simulink model "adcs_v15_integral_29april17"  (R2015b)
settings: Solver=ode4  StartTime=0.0  StopTime=20  FixedStep=s_SIM_STEP_SIZE  RelTol=1e-3
values from neighbouring files (symbols this model uses):
  A = ((T_SIDE + .29)*1e-3)^2    [constants_v13.m]    (also in constants_v15.m; constants_v15_Pow.m; constants_v15_Pow_ss_error.m; constants_v16_integral_kartavya.m)
  Ca_Solar_Drag = 1.4    [constants_v13.m]    (also in constants_v15.m = 0; constants_v15_Pow.m; constants_v15_Pow_ss_error.m; constants_v16_integral_kartavya.m)
  Cd = 2.2    [constants_v13.m]    (also in constants_v15.m = 0; constants_v15_Pow.m; constants_v15_Pow_ss_error.m; constants_v16_integral_kartavya.m)
  check_time = 60000    [constants_v13.m]    (also in constants_v15.m = 10000; constants_v15_Pow_ss_error.m = 10000; constants_v16_integral_kartavya.m = 10000; constants_v16_integral_light_sun_sgp_igrf_power_13Dec2011.m = 10000)
  equinox = datenum('21-Mar-2010 12:0:0')    [constants_v13.m]    (also in constants_v15.m; constants_v15_Pow.m = datenum('20-Mar-2015 12:0:0'); constants_v15_Pow_ss_error.m; constants_v16_integral_kartavya.m)
  I_MAX = 0.5    [constants_v13.m]    (also in constants_v15.m; constants_v15_Pow.m; constants_v15_Pow_ss_error.m; constants_v16_integral_kartavya.m)
  I_TORQUER = 3.6 / 7.31    (= 0.492476060192)    [constants_v13.m]    (also in constants_v15.m = 0.272727272727; constants_v15_Pow.m; constants_v15_Pow_ss_error.m; constants_v16_integral_kartavya.m)
  Kd = 2* m_INERTIA / (s_numOrbits * T_ORBIT )    [constants_v13.m]    (also in constants_v15.m = m_INERTIA * (2 + delta)* zeta * w; constants_v15_Pow.m = m_INERTIA * (2 + delta)* zeta * w; constants_v15_Pow_ss_error.m = m_INERTIA * (2 + delta)* zeta * w; constants_v16_integral_kartavya.m = m_INERTIA * (2 + delta)* zeta * w)
  Kdetumb = K_det*eye(3)    [constants_v13.m]    (also in constants_v15.m; constants_v15_Pow.m; constants_v15_Pow_ss_error.m; constants_v16_integral_kartavya.m)
  Ki = m_INERTIA * delta * zeta * w^3    [constants_v15.m]    (also in constants_v15_Pow.m; constants_v15_Pow_ss_error.m; constants_v16_integral_kartavya.m; constants_v16_integral_light_sun_sgp_igrf_power_13Dec2011.m)
  Kp = m_INERTIA / (s_numOrbits * T_ORBIT * zeta)^2    [constants_v13.m]    (also in constants_v15.m = m_INERTIA * (w*w + 2*delta*zeta^2*w^2); constants_v15_Pow.m = m_INERTIA * (w*w + 2*delta*zeta^2*w^2); constants_v15_Pow_ss_error.m = m_INERTIA * (w*w + 2*delta*zeta^2*w^2); constants_v16_integral_kartavya.m = m_INERTIA * (w*w + 2*delta*zeta^2*w^2))
  m_INERTIA = [Ixx Ixy Ixz; Ixy Iyy Iyz; Ixz Iyz Izz]    [constants_v13.m]    (also in constants_v15.m; constants_v15_Pow.m = 1*[Ixx Ixy Ixz; Ixy Iyy Iyz; Ixz Iyz Izz]; constants_v15_Pow_ss_error.m = 1*[Ixx Ixy Ixz; Ixy Iyy Iyz; Ixz Iyz Izz]; constants_v16_integral_kartavya.m)
  mu = 6.673e-11*5.9742e24    (= 398658366000000)    [constants_v13.m]    (also in constants_v15.m; constants_v15_Pow.m; constants_v15_Pow_ss_error.m; constants_v16_integral_kartavya.m)
  N = 40    [constants_v13.m]    (also in constants_v15.m = 60; constants_v15_Pow.m; constants_v15_Pow_ss_error.m; constants_v16_integral_kartavya.m)
  P_momentum_flux_from_the_sun = 4.4e-6    (= 4.4e-06)    [constants_v13.m]    (also in constants_v15.m = 0; constants_v15_Pow.m; constants_v15_Pow_ss_error.m; constants_v16_integral_kartavya.m)
  q_BI0 = x_fromEnvModel(1:4)'    [OILS_script.m]    (also in OILS_script_OBC_preflight_bounce_back.m; OILS_script_extended.m; OILS_script_preflight_test.m; constants_v13.m = euler2qBI(roll0,pitch0,yaw0))
  s_FRAME_SIZE = 2    [constants_v13.m]    (also in constants_v15.m; constants_v15_Pow.m; constants_v15_Pow_ss_error.m; constants_v16_integral_kartavya.m)
  s_m_MAX = 0.95    [constants_v13.m]    (also in constants_v15.m; constants_v15_Pow.m; constants_v15_Pow_ss_error.m; constants_v16_integral_kartavya.m)
  s_MAG_B = 2.5e-5    (= 2.5e-05)    [constants_v13.m]    (also in constants_v15.m; constants_v15_Pow.m; constants_v15_Pow_ss_error.m; constants_v16_integral_kartavya.m)
  s_MAGMETER_WEIGHT = .9    (= 0.9)    [constants_v13.m]    (also in constants_v15.m; constants_v15_Pow.m; constants_v15_Pow_ss_error.m; constants_v16_integral_kartavya.m)
  s_SIM_STEP_SIZE = 0.1    [constants_v13.m]    (also in constants_v15.m; constants_v15_Pow.m; constants_v15_Pow_ss_error.m; constants_v16_integral_kartavya.m)
  s_SS_ADC_gain = 5    [constants_v13.m]    (also in constants_v15.m = 3.3; constants_v15_Pow.m; constants_v15_Pow_ss_error.m; constants_v16_integral_kartavya.m)
  s_SS_ADC_res = 2^12 - 1    (= 4095)    [constants_v13.m]    (also in constants_v15.m = 1023; constants_v15_Pow.m; constants_v15_Pow_ss_error.m; constants_v16_integral_kartavya.m)
  s_SS_MAX_ANGLE = 85    [constants_v13.m]    (also in constants_v15.m = 55; constants_v15_Pow.m; constants_v15_Pow_ss_error.m; constants_v16_integral_kartavya.m)
  s_TAU_W = 60    [constants_v13.m]    (also in constants_v15.m; constants_v15_Pow.m; constants_v15_Pow_ss_error.m; constants_v16_integral_kartavya.m)
  s_x_MAGMETER_BIAS = 50e-9    (= 5e-08)    [constants_v13.m]    (also in constants_v15.m = 0; constants_v15_Pow.m; constants_v15_Pow_ss_error.m; constants_v16_integral_kartavya.m)
  side = 0.26    [constants_v13.m]    (also in constants_v15.m; constants_v15_Pow.m; constants_v15_Pow_ss_error.m; constants_v16_integral_kartavya.m)
  Snum = 6    [constants_v13.m]    (also in constants_v15.m; constants_v15_Pow.m; constants_v15_Pow_ss_error.m; constants_v16_integral_kartavya.m)
  TLE_epoch = datenum('18-Oct-2015 10:30:0')    [constants_v15.m]    (also in constants_v16_integral_kartavya.m = datenum('18-Oct-2010 10:30:0'); constants_v16_integral_light_sun_sgp_igrf_power_13Dec2011.m = datenum('18-Oct-2010 10:30:0'); precalcs.m)
  today = datenum('18-Oct-2010 10:30:0')    [constants_v13.m]    (also in constants_v15.m; constants_v15_Pow.m = datenum('18-Oct-2015 10:30:0'); constants_v15_Pow_ss_error.m; constants_v16_integral_kartavya.m)
  tol_q4 = 0.7    [constants_v13.m]    (also in constants_v15.m = 0.85; constants_v15_Pow.m = 0.85; constants_v15_Pow_ss_error.m = 0.85; constants_v16_integral_kartavya.m = 0.85)
  tol_w = 4e-3    (= 0.004)    [constants_v13.m]    (also in constants_v15.m; constants_v15_Pow.m; constants_v15_Pow_ss_error.m; constants_v16_integral_kartavya.m)
  tolw_n2d = 10e-3    (= 0.01)    [constants_v15.m]    (also in constants_v15_Pow.m = 0.008; constants_v15_Pow_ss_error.m; constants_v16_integral_kartavya.m; constants_v16_integral_light_sun_sgp_igrf_power_13Dec2011.m)
  Ts_display = 6    [constants_v13.m]    (also in constants_v15.m = 2; constants_v15_Pow.m; constants_v15_Pow_ss_error.m; constants_v16_integral_kartavya.m)
  v_COM_to_COP_b = [.2; 1.75; .2]*1e-2    [constants_v13.m]    (also in constants_v15.m = [.2; 1.75; .2]*0e-2; constants_v15_Pow.m; constants_v15_Pow_ss_error.m; constants_v16_integral_kartavya.m)
  v_S1 = [1 0 0]    [constants_v13.m]    (also in constants_v15.m; constants_v15_Pow.m; constants_v15_Pow_ss_error.m; constants_v16_integral_kartavya.m)
  v_S2 = [-1 0 0]    [constants_v13.m]    (also in constants_v15.m; constants_v15_Pow.m; constants_v15_Pow_ss_error.m; constants_v16_integral_kartavya.m)
  v_S3 = [0 1 0]    [constants_v13.m]    (also in constants_v15.m; constants_v15_Pow.m; constants_v15_Pow_ss_error.m; constants_v16_integral_kartavya.m)
  v_S4 = [0 -1 0]    [constants_v13.m]    (also in constants_v15.m; constants_v15_Pow.m; constants_v15_Pow_ss_error.m; constants_v16_integral_kartavya.m)
  v_S5 = [0 0 1]    [constants_v13.m]    (also in constants_v15.m; constants_v15_Pow.m; constants_v15_Pow_ss_error.m; constants_v16_integral_kartavya.m)
  v_S6 = [0 0 -1]    [constants_v13.m]    (also in constants_v15.m; constants_v15_Pow.m; constants_v15_Pow_ss_error.m; constants_v16_integral_kartavya.m)
  v_x_MOUNTING_THETA_ZYX_BODY_TORQUER = [1; 1; 1]* pi/180    [constants_v13.m]    (also in constants_v15.m; constants_v15_Pow.m; constants_v15_Pow_ss_error.m; constants_v16_integral_kartavya.m)
  wx0 = x_fromEnvModel(5)    [OILS_script.m]    (also in OILS_script_OBC_preflight_bounce_back.m; OILS_script_extended.m; OILS_script_preflight_test.m; constants_v13.m = 0.0349065850399)
  wy0 = x_fromEnvModel(6)    [OILS_script.m]    (also in OILS_script_OBC_preflight_bounce_back.m; OILS_script_extended.m; OILS_script_preflight_test.m; constants_v13.m = 0.0174532925199)
  wz0 = x_fromEnvModel(7)    [OILS_script.m]    (also in OILS_script_OBC_preflight_bounce_back.m; OILS_script_extended.m; OILS_script_preflight_test.m; constants_v13.m = -0.0349065850399)
undefined symbols (not defined in the file or in its folder): Earth, WGS84
libraries: xpcutilitieslib x17, commnoisgen2 x14, aerolibutil x2, aerolibtransform2 x1
(part 1 of 2)
settings Model: SimulationMode=accelerator  ExtModeTrigDuration=100  Creator=Jaideep  LastModifiedBy=sat_lab
settings SolverCC: AutoInsertRateTranBlk=on
settings DataIOCC: ExternalInput=constants_v13  SaveFinalState=on  SaveFormat=Array  SignalLoggingSaveFormat=ModelDataLogs  SaveOutput=off  SaveState=on  StateSaveName=tmp_raccel_xout
settings OptimizationCC: ExpressionDepthLimit=2147483647  EfficientMapNaN2IntZero=off
settings DebuggingCC: UnderspecifiedInitializationDetection=Classic  MergeDetectMultiDrivingBlocksExec=none  SolverPrmCheckMsg=warning  FcnCallInpInsideContextMsg=UseLocalSettings  StateNameClashWarn=warning
settings HardwareCC: ProdBitPerPointer=32  ProdLargestAtomicFloat=None  ProdIntDivRoundTo=Undefined  ProdEndianess=Unspecified  ProdWordSize=32  ProdHWDeviceType=32-bit Generic  TargetBitPerPointer=64  TargetLongLongMode=on  TargetIntDivRoundTo=Zero  TargetEndianess=LittleEndian  TargetWordSize=64  TargetHWDeviceType=MATLAB Host  ProdEqTarget=off
settings SFSimCC: SimParseCustomCode=off
settings RTWCC: SystemTargetFile=raccel.tlc  TemplateMakefile=raccel_default_tmf  RTWVerbose=off
settings CodeAppCC: GenerateComments=off  MaxIdLength=128  SimulinkBlockComments=off
settings RaccelTargetCC: ERTMultiwordTypeDef=System defined  ERTMultiwordLength=256  ParMdlRefBuildCompliant=off  GeneratePreprocessorConditionals=Disable all  ERTFirstTimeCompliant=off  MultiInstanceERTCode=off  ENABLE_SLEXEC_SSBRIDGE=0  RTWCAPIParams=on
settings ConfigComp: CovModelRefEnable=Off

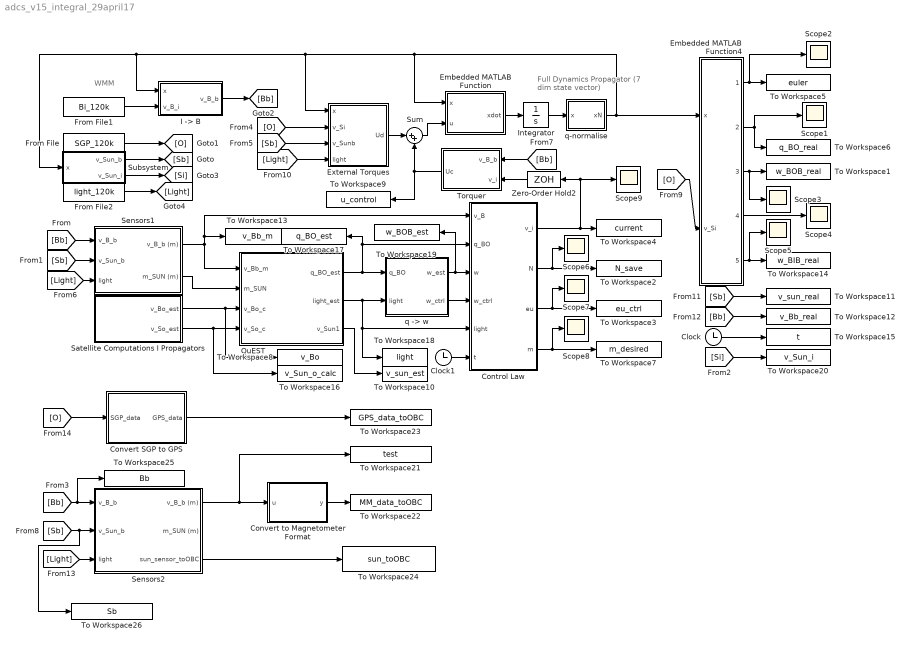
== system adcs_v15_integral_29april17 ==
  note: Full Dynamics Propagator
      |  (7 dim state vector)
  note: WMM
  Clock : Clock
  Clock1 : Clock
  Control Law : Subsystem  TreatAsAtomicUnit=on  SystemSampleTime=s_FRAME_SIZE
  Convert SGP to GPS : Subsystem
  Convert to Magnetometer Format : MATLAB Function  TreatAsAtomicUnit=on
  Embedded MATLAB Function : MATLAB Function  TreatAsAtomicUnit=on
  Embedded MATLAB Function4 : MATLAB Function  TreatAsAtomicUnit=on
  External Torques : Subsystem
  From File : FromFile  FileName=SGP_120k
  From File1 : FromFile  FileName=Bi_120k
  From File2 : FromFile  FileName=light_120k  SampleTime=0
  "I -> B" : Subsystem
  Integrator : Integrator  InitialCondition=[q_BI0; wx0; wy0; wz0]
  QuEST : MATLAB Function  TreatAsAtomicUnit=on  SystemSampleTime=s_FRAME_SIZE
  Satellite Computations I Propagators : Subsystem  TreatAsAtomicUnit=on  SystemSampleTime=s_FRAME_SIZE
  Scope{1..9} (9 alike) : Scope
  Sensors1 : Subsystem
  Sensors2 : Subsystem
  Subsystem : Subsystem
  Sum : Sum  Inputs=|++
  To Workspace1 : ToWorkspace  VariableName=w_BOB_real  SampleTime=Ts_display
  To Workspace10 : ToWorkspace  VariableName=v_sun_est  SampleTime=Ts_display
  To Workspace11 : ToWorkspace  VariableName=v_sun_real  SampleTime=Ts_display
  To Workspace12 : ToWorkspace  VariableName=v_Bb_real  SampleTime=Ts_display
  To Workspace13 : ToWorkspace  VariableName=v_Bb_m  SampleTime=Ts_display
  To Workspace14 : ToWorkspace  VariableName=w_BIB_real  SampleTime=Ts_display
  To Workspace15 : ToWorkspace  VariableName=t  SampleTime=Ts_display
  To Workspace16 : ToWorkspace  VariableName=v_Sun_o_calc  SampleTime=Ts_display
  To Workspace17 : ToWorkspace  VariableName=q_BO_est  SampleTime=Ts_display
  To Workspace18 : ToWorkspace  VariableName=light  SampleTime=Ts_display
  To Workspace19 : ToWorkspace  VariableName=w_BOB_est  SampleTime=Ts_display
  To Workspace2 : ToWorkspace  VariableName=N_save  SampleTime=Ts_display
  To Workspace20 : ToWorkspace  VariableName=v_Sun_i  SampleTime=Ts_display
  To Workspace21 : ToWorkspace  VariableName=test  SampleTime=-1
  To Workspace22 : ToWorkspace  VariableName=MM_data_toOBC  SampleTime=Ts_display
  To Workspace23 : ToWorkspace  VariableName=GPS_data_toOBC  SampleTime=Ts_display
  To Workspace24 : ToWorkspace  VariableName=sun_toOBC  SampleTime=Ts_display
  To Workspace25 : ToWorkspace  VariableName=Bb  SampleTime=-1
  To Workspace26 : ToWorkspace  VariableName=Sb  SampleTime=-1
  To Workspace3 : ToWorkspace  VariableName=eu_ctrl  SampleTime=Ts_display
  To Workspace4 : ToWorkspace  VariableName=current  SampleTime=Ts_display
  To Workspace5 : ToWorkspace  VariableName=euler  SampleTime=Ts_display
  To Workspace6 : ToWorkspace  VariableName=q_BO_real  SampleTime=Ts_display
  To Workspace7 : ToWorkspace  VariableName=m_desired  SampleTime=Ts_display
  To Workspace8 : ToWorkspace  VariableName=v_Bo  SampleTime=Ts_display
  To Workspace9 : ToWorkspace  VariableName=u_control  SampleTime=Ts_display
  Torquer : Subsystem
  Zero-Order Hold2 : ZeroOrderHold  SampleTime=s_FRAME_SIZE
  "q -> w" : Subsystem  TreatAsAtomicUnit=on  SystemSampleTime=s_FRAME_SIZE
  q-normalise : MATLAB Function  TreatAsAtomicUnit=on
  wires:
  Embedded MATLAB Function/1(xdot) -> Integrator/1
  Integrator/1 -> q-normalise/1(x)
  From File/1 -> [O]
  q-normalise/1(xN) -> Subsystem/1(x), "I -> B"/1(x), External Torques/1(x), Embedded MATLAB Function/1(x), Embedded MATLAB Function4/1(x)
  Sum/1 -> Embedded MATLAB Function/2(u)
  "I -> B"/1(v_B_b) -> [Bb]
  Subsystem/1(v_Sun_b) -> [Sb]
  [Bb] -> Sensors1/1(v_B_b)
  [Sb] -> Sensors1/2(v_Sun_b)
  Subsystem/2(v_Sun_i) -> [Si]
  [O] -> External Torques/2(v_Si)
  [Sb] -> External Torques/3(v_Sunb)
  [Bb] -> Torquer/1(v_B_b)
  [Light] -> Sensors1/3(light)
  Sensors1/2(m_SUN (m)) -> QuEST/2(m_SUN)
  Sensors1/1(v_B_b (m)) -> QuEST/1(v_Bb_m), Control Law/1(v_B), To Workspace13/1
  Zero-Order Hold2/1 -> Torquer/2(v_i)
  Torquer/1(Uc) -> Sum/2, To Workspace9/1
  Satellite Computations I Propagators/1(v_Bo_est) -> To Workspace8/1, QuEST/3(v_Bo_c)
  Satellite Computations I Propagators/2(v_So_est) -> To Workspace16/1, QuEST/4(v_So_c)
  QuEST/1(q_BO_est) -> "q -> w"/1(q_BO), Control Law/2(q_BO), To Workspace17/1
  QuEST/2(light_est) -> "q -> w"/2(light), Control Law/5(light), To Workspace18/1
  Control Law/1(v_i) -> To Workspace4/1, Zero-Order Hold2/1, Scope9/1
  [O] -> Embedded MATLAB Function4/2(v_Si)
  Control Law/2(N) -> To Workspace2/1, Scope6/1
  From File2/1 -> [Light]
  Control Law/3(eu) -> To Workspace3/1, Scope7/1
  Control Law/4(m) -> To Workspace7/1, Scope8/1
  "q -> w"/1(w_est) -> Control Law/3(w), To Workspace19/1
  [Light] -> External Torques/4(light)
  "q -> w"/2(w_ctrl) -> Control Law/4(w_ctrl)
  QuEST/3(v_Sun1) -> To Workspace10/1
  [Sb] -> To Workspace11/1
  [Bb] -> To Workspace12/1
  Clock/1 -> To Workspace15/1
  From File1/1 -> "I -> B"/2(v_B_i)
  Clock1/1 -> Control Law/6(t)
  Embedded MATLAB Function4/3(w_BOB) -> To Workspace1/1, Scope3/1
  Embedded MATLAB Function4/2(q_BO) -> To Workspace6/1, Scope1/1
  Embedded MATLAB Function4/1(euler) -> To Workspace5/1, Scope2/1
  Embedded MATLAB Function4/5(w_BIB) -> To Workspace14/1, Scope5/1
  Embedded MATLAB Function4/4(modw) -> Scope4/1
  [Si] -> To Workspace20/1
  External Torques/1(Ud) -> Sum/1
  [O] -> Convert SGP to GPS/1(SGP_data)
  Convert SGP to GPS/1(GPS_data) -> To Workspace23/1
  Convert to Magnetometer Format/1(y) -> To Workspace22/1
  [Bb] -> To Workspace25/1, Sensors2/1(v_B_b)
  [Sb] -> To Workspace26/1, Sensors2/2(v_Sun_b)
  [Light] -> Sensors2/3(light)
  Sensors2/3(sun_sensor_toOBC) -> To Workspace24/1
  Sensors2/1(v_B_b (m)) -> To Workspace21/1, Convert to Magnetometer Format/1(u)

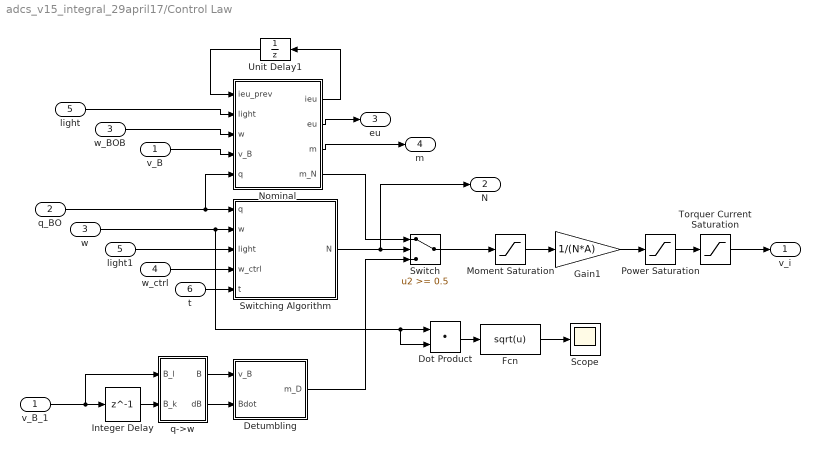
== system adcs_v15_integral_29april17/Control Law ==
  v_B : Inport
  q_BO : Inport  Port=2
  w : Inport  Port=3
  w_ctrl : Inport  Port=4
  light : Inport  Port=5
  t : Inport  Port=6
  Detumbling : MATLAB Function  TreatAsAtomicUnit=on
  Dot Product : DotProduct  InputSameDT=on  OutDataTypeStr=Inherit: Inherit via internal rule
  Fcn : Fcn  Expr=sqrt(u)
  Gain1 : Gain  Gain=1/(N*A)
  Integer Delay : Delay  DelayLength=1  InputProcessing=Inherited
  Moment Saturation : Saturate  UpperLimit=s_m_MAX  LowerLimit=-s_m_MAX
  Nominal : MATLAB Function  TreatAsAtomicUnit=on
  Power Saturation : Saturate  UpperLimit=I_MAX  LowerLimit=-I_MAX
  Scope : Scope
  Switch : Switch  Threshold=0.5
  Switching Algorithm : Subsystem
  Torquer Current Saturation : Saturate  UpperLimit=I_TORQUER  LowerLimit=-I_TORQUER
  Unit Delay1 : UnitDelay  InitialCondition=[0;0;0]  SampleTime=-1
  light1 : InportShadow  Port=5
  q->w : MATLAB Function  TreatAsAtomicUnit=on
  v_B_1 : InportShadow
  w_BOB : InportShadow  Port=3
  v_i : Outport
  N : Outport  Port=2
  eu : Outport  Port=3
  m : Outport  Port=4
  wires:
  w_ctrl/1 -> Switching Algorithm/4(w_ctrl)
  Nominal/3(m) -> m/1
  Nominal/2(eu) -> eu/1
  w_BOB/1 -> Nominal/3(w)
  light1/1 -> Switching Algorithm/3(light)
  v_B/1 -> Nominal/4(v_B)
  q->w/2(dB) -> Detumbling/2(Bdot)
  v_B_1/1 -> Integer Delay/1, q->w/1(B_l)
  w/1 -> Switching Algorithm/2(w), Dot Product/1, Dot Product/2
  Nominal/4(m_N) -> Switch/1
  Switching Algorithm/1(N) -> Switch/2, N/1
  Detumbling/1(m_D) -> Switch/3
  Switch/1 -> Moment Saturation/1
  Power Saturation/1 -> Torquer Current Saturation/1
  Moment Saturation/1 -> Gain1/1
  Torquer Current Saturation/1 -> v_i/1
  Gain1/1 -> Power Saturation/1
  light/1 -> Nominal/2(light)
  q_BO/1 -> Switching Algorithm/1(q), Nominal/5(q)
  Integer Delay/1 -> q->w/2(B_k)
  q->w/1(B) -> Detumbling/1(v_B)
  t/1 -> Switching Algorithm/5(t)
  Dot Product/1 -> Fcn/1
  Fcn/1 -> Scope/1
  Unit Delay1/1 -> Nominal/1(ieu_prev)
  Nominal/1(ieu) -> Unit Delay1/1

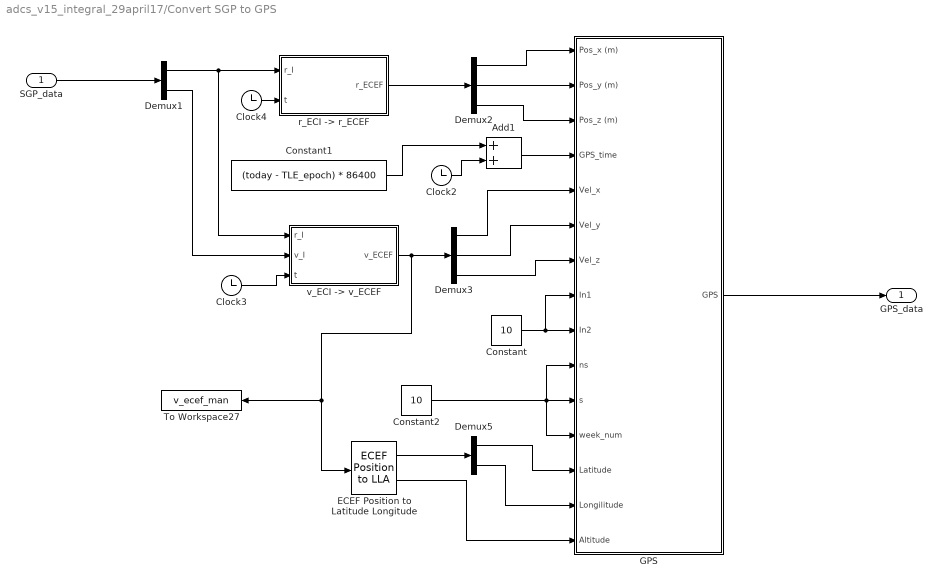
== system adcs_v15_integral_29april17/Convert SGP to GPS ==
  SGP_data : Inport
  Add1 : Sum
  Clock2 : Clock
  Clock3 : Clock
  Clock4 : Clock
  Constant : Constant  Value=10  OutDataTypeStr=uint8
  Constant1 : Constant  Value=(today - TLE_epoch) * 86400  VectorParams1D=off
  Constant2 : Constant  Value=10  OutDataTypeStr=double
  Demux1 : Demux  Outputs=2
  Demux2 : Demux  Outputs=3
  Demux3 : Demux  Outputs=3
  Demux5 : Demux  Outputs=2
  ECEF Position to Latitude Longitude : aerolibtransform2/ECEF Position to LLA  units=Metric (MKS)  ptype=Earth (WGS84)  F=1/298.257223563  R=6378137
  GPS : Subsystem
  To Workspace27 : ToWorkspace  VariableName=v_ecef_man  SampleTime=Ts_display
  "r_ECI -> r_ECEF" : MATLAB Function  TreatAsAtomicUnit=on
  "v_ECI -> v_ECEF" : MATLAB Function  TreatAsAtomicUnit=on
  GPS_data : Outport
  wires:
  Constant/1 -> GPS/9(In2), GPS/8(In1)
  ECEF Position to Latitude Longitude/1 -> Demux5/1
  ECEF Position to Latitude Longitude/2 -> GPS/15(Altitude)
  Constant2/1 -> GPS/10(ns), GPS/12(week_num), GPS/11(s)
  Demux5/1 -> GPS/13(Latitude)
  GPS/1(GPS) -> GPS_data/1
  Demux5/2 -> GPS/14("Longilitude ")
  Constant1/1 -> Add1/1
  Clock2/1 -> Add1/2
  Add1/1 -> GPS/4(GPS_time)
  Demux1/2 -> "v_ECI -> v_ECEF"/2(v_I)
  "v_ECI -> v_ECEF"/1(v_ECEF) -> Demux3/1, ECEF Position to Latitude Longitude/1, To Workspace27/1
  Demux3/1 -> GPS/5(Vel_x)
  Demux3/2 -> GPS/6(Vel_y)
  Clock3/1 -> "v_ECI -> v_ECEF"/3(t)
  Demux3/3 -> GPS/7(Vel_z)
  "r_ECI -> r_ECEF"/1(r_ECEF) -> Demux2/1
  Demux2/1 -> GPS/1(Pos_x (m))
  Demux2/2 -> GPS/2(Pos_y (m))
  Demux2/3 -> GPS/3(Pos_z (m))
  Demux1/1 -> "v_ECI -> v_ECEF"/1(r_I), "r_ECI -> r_ECEF"/1(r_I)
  SGP_data/1 -> Demux1/1
  Clock4/1 -> "r_ECI -> r_ECEF"/2(t)

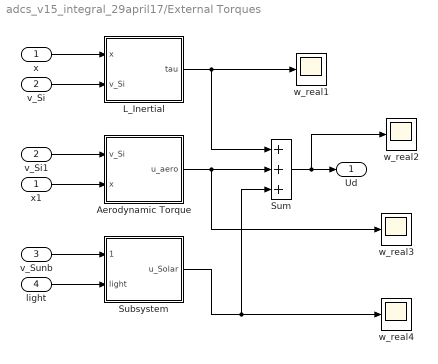
== system adcs_v15_integral_29april17/External Torques ==
  x : Inport
  v_Si : Inport  Port=2
  v_Sunb : Inport  Port=3
  light : Inport  Port=4
  Aerodynamic Torque : Subsystem
  L_Inertial : MATLAB Function  TreatAsAtomicUnit=on
  Subsystem : Subsystem
  Sum : Sum  Inputs=+++
  v_Si1 : InportShadow  Port=2
  w_real{1..4} (4 alike) : Scope
  x1 : InportShadow
  Ud : Outport
  wires:
  x/1 -> L_Inertial/1(x)
  v_Si/1 -> L_Inertial/2(v_Si)
  L_Inertial/1(tau) -> Sum/1, w_real1/1
  Aerodynamic Torque/1(u_aero) -> Sum/2, w_real3/1
  x1/1 -> Aerodynamic Torque/2(x)
  v_Si1/1 -> Aerodynamic Torque/1(v_Si)
  Sum/1 -> Ud/1, w_real2/1
  v_Sunb/1 -> Subsystem/1(v_Sun_b)
  Subsystem/1(u_Solar) -> Sum/3, w_real4/1
  light/1 -> Subsystem/2(light)

== system adcs_v15_integral_29april17/I -> B ==
  x : Inport
  v_B_i : Inport  Port=2
  Gain : Gain  Gain=1e-9
  L_Inertial : MATLAB Function  TreatAsAtomicUnit=on
  v_B_b : Outport
  wires:
  L_Inertial/1(v_B) -> v_B_b/1
  x/1 -> L_Inertial/1(x)
  v_B_i/1 -> Gain/1
  Gain/1 -> L_Inertial/2(v_I)

== system adcs_v15_integral_29april17/Satellite Computations I Propagators ==
  From File : FromFile  FileName=Si_120k
  From File2 : FromFile  FileName=SGP_est_120k
  From File3 : FromFile  FileName=Bi8_est_120k
  m_TOI_NEW : MATLAB Function  TreatAsAtomicUnit=on
  m_TOI_NEW1 : MATLAB Function  TreatAsAtomicUnit=on
  v_Bo_est : Outport
  v_So_est : Outport  Port=2
  wires:
  From File3/1 -> m_TOI_NEW/2(v_I)
  From File2/1 -> m_TOI_NEW1/2(ECI), m_TOI_NEW/1(ECI)
  From File/1 -> m_TOI_NEW1/1(v_I)
  m_TOI_NEW/1(v_O) -> v_Bo_est/1
  m_TOI_NEW1/1(v_O) -> v_So_est/1

== system adcs_v15_integral_29april17/Sensors1 ==
  note: 'm' stands for measured
  v_B_b : Inport
  v_Sun_b : Inport  Port=2
  light : Inport  Port=3
  Magnetometer simple : Subsystem
  Sun Sensors : Subsystem
  v_B_b (m) : Outport
  m_SUN (m) : Outport  Port=2
  wires:
  light/1 -> Sun Sensors/2(Light)
  Magnetometer simple/1(v_B_b(m)) -> v_B_b (m)/1
  v_B_b/1 -> Magnetometer simple/1(v_B_b)
  v_Sun_b/1 -> Sun Sensors/1(v_Sun_b)
  Sun Sensors/1(m_SUN) -> m_SUN (m)/1

== system adcs_v15_integral_29april17/Sensors2 ==
  note: 'm' stands for measured
  v_B_b : Inport
  v_Sun_b : Inport  Port=2
  light : Inport  Port=3
  Magnetometer simple : Subsystem
  Sun Sensors : Subsystem
  v_B_b (m) : Outport
  m_SUN (m) : Outport  Port=2
  sun_sensor_toOBC : Outport  Port=3
  wires:
  light/1 -> Sun Sensors/2(Light)
  Magnetometer simple/1(v_B_b(m)) -> v_B_b (m)/1
  v_B_b/1 -> Magnetometer simple/1(v_B_b)
  v_Sun_b/1 -> Sun Sensors/1(v_Sun_b)
  Sun Sensors/1(m_SUN) -> m_SUN (m)/1
  Sun Sensors/2(sun_sensor_toOBC) -> sun_sensor_toOBC/1

== system adcs_v15_integral_29april17/Subsystem ==
  x : Inport
  From File : FromFile  FileName=Si_120k  SampleTime=0
  f: I->B : MATLAB Function  TreatAsAtomicUnit=on
  v_Sun_b : Outport
  v_Sun_i : Outport  Port=2
  wires:
  x/1 -> f: I->B/1(x)
  f: I->B/1(v_B) -> v_Sun_b/1
  From File/1 -> f: I->B/2(v_I), v_Sun_i/1

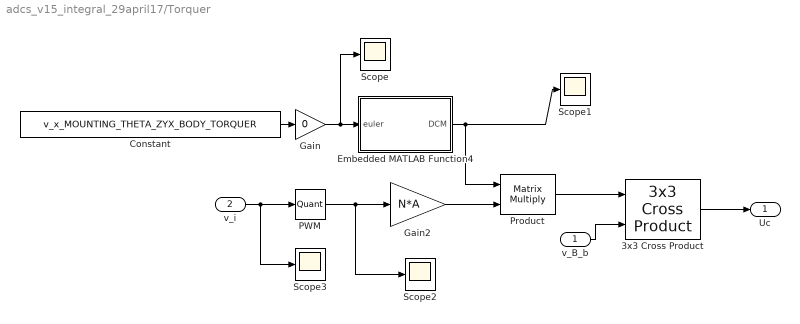
== system adcs_v15_integral_29april17/Torquer ==
  v_B_b : Inport
  v_i : Inport  Port=2
  3x3 Cross Product : aerolibutil/3x3 Cross Product
  Constant : Constant  Value=v_x_MOUNTING_THETA_ZYX_BODY_TORQUER
  Embedded MATLAB Function4 : MATLAB Function  TreatAsAtomicUnit=on
  Gain : Gain  Gain=0
  Gain2 : Gain  Gain=N*A
  PWM : Quantizer  QuantizationInterval=s_PWM_RES
  Product : Product  Multiplication=Matrix(*)  RndMeth=Zero
  Scope{,1..3} (4 alike) : Scope
  Uc : Outport
  wires:
  PWM/1 -> Gain2/1, Scope2/1
  v_B_b/1 -> 3x3 Cross Product/2
  3x3 Cross Product/1 -> Uc/1
  v_i/1 -> PWM/1, Scope3/1
  Embedded MATLAB Function4/1(DCM) -> Product/1, Scope1/1
  Gain2/1 -> Product/2
  Product/1 -> 3x3 Cross Product/1
  Constant/1 -> Gain/1
  Gain/1 -> Embedded MATLAB Function4/1(euler), Scope/1

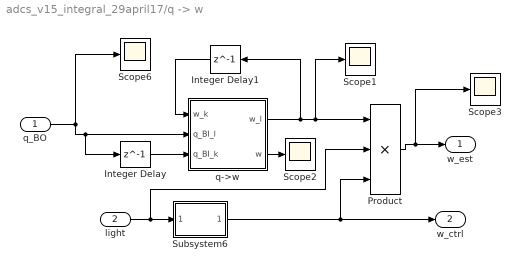
== system adcs_v15_integral_29april17/q -> w ==
  q_BO : Inport
  light : Inport  Port=2
  Integer Delay : Delay  DelayLength=1  InputProcessing=Inherited
  Integer Delay1 : Delay  DelayLength=1  InitialCondition=[0;0;0]  InputProcessing=Inherited
  Product : Product  Inputs=3  RndMeth=Zero
  Scope{1..3,6} (4 alike) : Scope
  Subsystem6 : Subsystem
  q->w : MATLAB Function  TreatAsAtomicUnit=on
  w_est : Outport
  w_ctrl : Outport  Port=2
  wires:
  Subsystem6/1(w-ctrl) -> w_ctrl/1, Product/3
  q_BO/1 -> Integer Delay/1, q->w/2(q_BI_l), Scope6/1
  light/1 -> Product/2, Subsystem6/1(light)
  Product/1 -> w_est/1, Scope3/1
  Integer Delay/1 -> q->w/3(q_BI_k)
  q->w/1(w_l) -> Integer Delay1/1, Product/1, Scope1/1
  Integer Delay1/1 -> q->w/1(w_k)
  q->w/2(w) -> Scope2/1

== system adcs_v15_integral_29april17/Control Law/Switching Algorithm ==
  note: remov the t=0 checking
      | code, not necessary
  q : Inport
  w : Inport  Port=2
  light : Inport  Port=3
  w_ctrl : Inport  Port=4
  t : Inport  Port=5
  Scope1 : Scope
  Unit Delay : UnitDelay  SampleTime=-1
  Unit Delay1 : UnitDelay  SampleTime=-1
  gate pulse : MATLAB Function  TreatAsAtomicUnit=on
  N : Outport
  wires:
  t/1 -> gate pulse/4(t)
  w_ctrl/1 -> gate pulse/6(w_ctrl)
  light/1 -> gate pulse/5(light_flag)
  gate pulse/1(N) -> N/1, Unit Delay1/1
  q/1 -> gate pulse/3(q)
  gate pulse/3(t_now) -> Unit Delay/1
  w/1 -> gate pulse/2(w)
  Unit Delay/1 -> gate pulse/7(t_now_prev)
  Unit Delay1/1 -> gate pulse/1(N_prev)
  gate pulse/2(P) -> Scope1/1

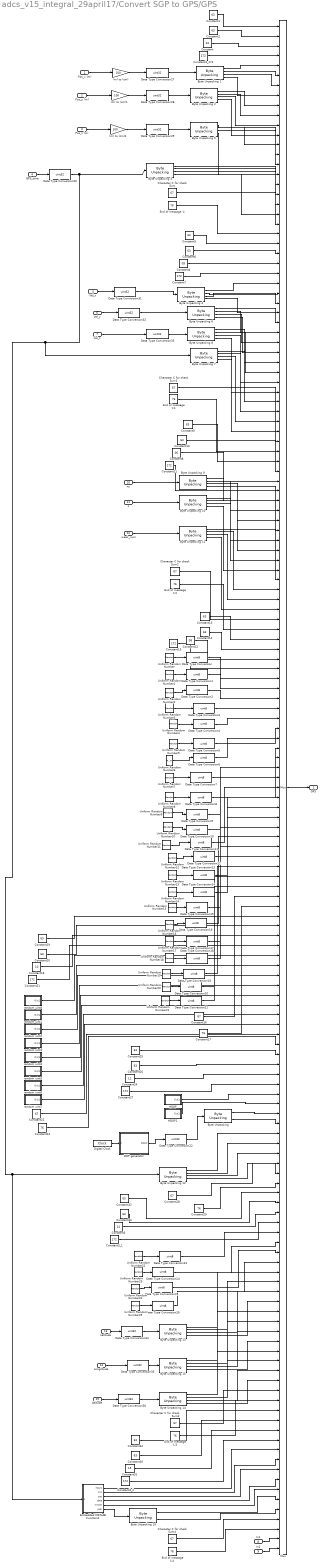
== system adcs_v15_integral_29april17/Convert SGP to GPS/GPS ==
  Pos_x (m) : Inport
  Pos_y (m) : Inport  Port=2
  Pos_z (m) : Inport  Port=3
  GPS_time : Inport  Port=4
  Vel_x : Inport  Port=5
  Vel_y : Inport  Port=6
  Vel_z : Inport  Port=7
  In1 : Inport  Port=8  OutDataTypeStr=uint8
  In2 : Inport  Port=9  OutDataTypeStr=uint8
  ns : Inport  Port=10
  s : Inport  Port=11
  week_num : Inport  Port=12
  Latitude : Inport  Port=13
  "Longilitude " : Inport  Port=14
  Altitude : Inport  Port=15
  (m) to (cm) : Gain  Gain=100  OutDataTypeStr=double
  (m) to (cm)1 : Gain  Gain=100
  (m) to (cm)2 : Gain  Gain=100
  Byte Unpacking {,1..16} (17 alike) : xpcutilitieslib/Byte Unpacking 
  Character C for check Sum{,1..4} (5 alike) : Constant  Value=67  OutDataTypeStr=uint8
  Constant : Constant  Value=04  OutDataTypeStr=uint8
  Constant{1..2,5..6,9..10,13..14,19..20,25..26,32..35} (16 alike) : Constant  Value=63  OutDataTypeStr=uint8
  Constant{7,11,15,21,27} (5 alike) : Constant  Value=172  OutDataTypeStr=uint8
  Constant12 : Constant  Value=08  OutDataTypeStr=uint8
  Constant16 : Constant  Value=67  OutDataTypeStr=uint8
  Constant17 : Constant  Value=76  OutDataTypeStr=uint8
  Constant18 : Constant  Value=10  OutDataTypeStr=uint8
  Constant22 : Constant  Value=67  OutDataTypeStr=uint8
  Constant23 : Constant  Value=76  OutDataTypeStr=uint8
  Constant24 : Constant  Value=11  OutDataTypeStr=uint8
  Constant28 : Constant  Value=67  OutDataTypeStr=uint8
  Constant29 : Constant  Value=76  OutDataTypeStr=uint8
  Constant3 : Constant  Value=14  OutDataTypeStr=uint8
  Constant31 : Constant  Value=15  OutDataTypeStr=uint8
  Constant3_1 : Constant  Value=172  OutDataTypeStr=uint8
  Constant3_172 : Constant  Value=172  OutDataTypeStr=uint8
  Constant3_2 : Constant  Value=172  OutDataTypeStr=uint8
  Constant4 : Constant  Value=05  OutDataTypeStr=uint8
  Constant8 : Constant  Value=06  OutDataTypeStr=uint8
  DOP generator : MATLAB Function  TreatAsAtomicUnit=on
  Data Type Conversion{,1..21,23..26} (26 alike) : DataTypeConversion  OutDataTypeStr=uint8
  Data Type Conversion{22,27..36} (11 alike) : DataTypeConversion  OutDataTypeStr=uint32
  Digital Clock : DigitalClock  SampleTime=0.1
  Embedded MATLAB Function2 : MATLAB Function  TreatAsAtomicUnit=on
  End of message 'L'{,1..4} (5 alike) : Constant  Value=76  OutDataTypeStr=uint8
  HDOP : Subsystem
  HDOP1 : Subsystem
  Mux : Mux  Inputs=155
  Uniform Random Number{,1..25} (26 alike) : UniformRandomNumber  Minimum=0  Maximum=256  Seed=1  SampleTime=0.1
  random uint1 : Subsystem
  random uint2 : Subsystem
  random uint3 : Subsystem
  random uint4 : Subsystem
  random uint5 : Subsystem
  random uint6 : Subsystem
  random uint7 : Subsystem
  random uint8 : Subsystem
  GPS : Outport
  wires:
  Constant1/1 -> Mux/1
  Constant2/1 -> Mux/2
  Constant/1 -> Mux/3
  Constant3_172/1 -> Mux/4
  GPS_time/1 -> Data Type Conversion30/1
  Byte Unpacking 3/1 -> Mux/17
  Byte Unpacking 3/2 -> Mux/18
  Byte Unpacking 3/3 -> Mux/19
  Character C for check Sum/1 -> Mux/21
  End of message 'L'/1 -> Mux/22
  Byte Unpacking 3/4 -> Mux/20
  Pos_x (m)/1 -> (m) to (cm)/1
  Pos_y (m)/1 -> (m) to (cm)1/1
  Pos_z (m)/1 -> (m) to (cm)2/1
  Byte Unpacking 5/1 -> Mux/13
  Byte Unpacking 5/2 -> Mux/14
  Byte Unpacking 5/3 -> Mux/15
  Byte Unpacking 5/4 -> Mux/16
  Byte Unpacking 1/1 -> Mux/5
  Byte Unpacking 1/2 -> Mux/6
  Byte Unpacking 1/3 -> Mux/7
  Byte Unpacking 1/4 -> Mux/8
  Byte Unpacking 2/1 -> Mux/9
  Byte Unpacking 2/2 -> Mux/10
  Byte Unpacking 2/3 -> Mux/11
  Byte Unpacking 2/4 -> Mux/12
  Constant5/1 -> Mux/23
  Constant6/1 -> Mux/24
  Constant4/1 -> Mux/25
  Constant7/1 -> Mux/26
  Byte Unpacking 4/1 -> Mux/27
  Byte Unpacking 4/2 -> Mux/28
  Byte Unpacking 4/3 -> Mux/29
  Byte Unpacking 4/4 -> Mux/30
  Byte Unpacking 6/1 -> Mux/31
  Byte Unpacking 6/2 -> Mux/32
  Byte Unpacking 6/3 -> Mux/33
  Byte Unpacking 6/4 -> Mux/34
  Byte Unpacking 8/1 -> Mux/35
  Byte Unpacking 8/2 -> Mux/36
  Byte Unpacking 8/3 -> Mux/37
  Byte Unpacking 8/4 -> Mux/38
  Byte Unpacking 7/1 -> Mux/39
  Byte Unpacking 7/2 -> Mux/40
  Byte Unpacking 7/3 -> Mux/41
  Byte Unpacking 7/4 -> Mux/42
  Character C for check Sum1/1 -> Mux/43
  End of message 'L'1/1 -> Mux/44
  Constant9/1 -> Mux/45
  Constant10/1 -> Mux/46
  Constant8/1 -> Mux/47
  Constant11/1 -> Mux/48
  Byte Unpacking 9/1 -> Mux/49
  Byte Unpacking 9/2 -> Mux/50
  Byte Unpacking 9/3 -> Mux/51
  Byte Unpacking 9/4 -> Mux/52
  Byte Unpacking 10/1 -> Mux/53
  Byte Unpacking 10/2 -> Mux/54
  Byte Unpacking 10/3 -> Mux/55
  Byte Unpacking 10/4 -> Mux/56
  Byte Unpacking 11/1 -> Mux/57
  Byte Unpacking 11/2 -> Mux/58
  Byte Unpacking 11/3 -> Mux/59
  Byte Unpacking 11/4 -> Mux/60
  Character C for check Sum2/1 -> Mux/61
  End of message 'L'2/1 -> Mux/62
  Uniform Random Number/1 -> Data Type Conversion/1
  Uniform Random Number1/1 -> Data Type Conversion1/1
  Uniform Random Number2/1 -> Data Type Conversion2/1
  Uniform Random Number3/1 -> Data Type Conversion3/1
  Uniform Random Number4/1 -> Data Type Conversion4/1
  Uniform Random Number5/1 -> Data Type Conversion5/1
  Uniform Random Number6/1 -> Data Type Conversion6/1
  Uniform Random Number7/1 -> Data Type Conversion7/1
  Uniform Random Number8/1 -> Data Type Conversion8/1
  Uniform Random Number9/1 -> Data Type Conversion9/1
  Uniform Random Number10/1 -> Data Type Conversion10/1
  Uniform Random Number11/1 -> Data Type Conversion11/1
  Uniform Random Number12/1 -> Data Type Conversion12/1
  Uniform Random Number13/1 -> Data Type Conversion13/1
  Uniform Random Number14/1 -> Data Type Conversion14/1
  Uniform Random Number15/1 -> Data Type Conversion15/1
  Uniform Random Number16/1 -> Data Type Conversion16/1
  Uniform Random Number17/1 -> Data Type Conversion17/1
  Uniform Random Number18/1 -> Data Type Conversion18/1
  Uniform Random Number19/1 -> Data Type Conversion19/1
  Uniform Random Number20/1 -> Data Type Conversion20/1
  Uniform Random Number21/1 -> Data Type Conversion21/1
  Constant13/1 -> Mux/63
  Constant14/1 -> Mux/64
  Constant12/1 -> Mux/65
  Constant15/1 -> Mux/66
  Data Type Conversion/1 -> Mux/67
  Data Type Conversion1/1 -> Mux/68
  Data Type Conversion2/1 -> Mux/69
  Data Type Conversion3/1 -> Mux/70
  Data Type Conversion4/1 -> Mux/71
  Data Type Conversion5/1 -> Mux/72
  Data Type Conversion6/1 -> Mux/73
  Data Type Conversion7/1 -> Mux/74
  Data Type Conversion8/1 -> Mux/75
  Data Type Conversion9/1 -> Mux/76
  Data Type Conversion10/1 -> Mux/77
  Data Type Conversion11/1 -> Mux/78
  Data Type Conversion12/1 -> Mux/79
  Data Type Conversion13/1 -> Mux/80
  Data Type Conversion14/1 -> Mux/81
  Data Type Conversion15/1 -> Mux/82
  Data Type Conversion16/1 -> Mux/83
  Data Type Conversion17/1 -> Mux/84
  Data Type Conversion18/1 -> Mux/85
  Data Type Conversion19/1 -> Mux/86
  Data Type Conversion20/1 -> Mux/87
  Data Type Conversion21/1 -> Mux/88
  Constant16/1 -> Mux/89
  Constant17/1 -> Mux/90
  Digital Clock/1 -> DOP generator/1(t)
  DOP generator/1(PDOP) -> Data Type Conversion22/1
  Data Type Conversion22/1 -> "Byte Unpacking "/1
  ns/1 -> Byte Unpacking 9/1
  s/1 -> Byte Unpacking 10/1
  week_num/1 -> Byte Unpacking 11/1
  Uniform Random Number22/1 -> Data Type Conversion23/1
  Uniform Random Number23/1 -> Data Type Conversion24/1
  Uniform Random Number24/1 -> Data Type Conversion25/1
  Uniform Random Number25/1 -> Data Type Conversion26/1
  Constant19/1 -> Mux/91
  Constant20/1 -> Mux/92
  Constant18/1 -> Mux/93
  Constant21/1 -> Mux/94
  random uint8/1(Out1) -> Mux/95
  random uint1/1(Out1) -> Mux/96
  random uint2/1(Out1) -> Mux/97
  random uint3/1(Out1) -> Mux/98
  random uint4/1(Out1) -> Mux/99
  random uint5/1(Out1) -> Mux/100
  random uint6/1(Out1) -> Mux/101
  random uint7/1(Out1) -> Mux/102
  Constant22/1 -> Mux/103
  Constant23/1 -> Mux/104
  Constant25/1 -> Mux/105
  Constant26/1 -> Mux/106
  Constant24/1 -> Mux/107
  Constant27/1 -> Mux/108
  HDOP/1(Out1) -> Mux/109
  HDOP1/1(Out1) -> Mux/110
  "Byte Unpacking "/1 -> Mux/111
  "Byte Unpacking "/2 -> Mux/112
  Byte Unpacking 12/1 -> Mux/113
  Byte Unpacking 12/2 -> Mux/114
  Byte Unpacking 12/3 -> Mux/115
  Byte Unpacking 12/4 -> Mux/116
  Constant28/1 -> Mux/117
  Constant29/1 -> Mux/118
  Constant32/1 -> Mux/119
  Constant33/1 -> Mux/120
  Constant3/1 -> Mux/121
  Constant3_1/1 -> Mux/122
  Data Type Conversion23/1 -> Mux/123
  Data Type Conversion24/1 -> Mux/124
  Data Type Conversion25/1 -> Mux/125
  Data Type Conversion26/1 -> Mux/126
  Byte Unpacking 13/1 -> Mux/127
  Byte Unpacking 13/2 -> Mux/128
  Byte Unpacking 13/3 -> Mux/129
  Byte Unpacking 13/4 -> Mux/130
  Byte Unpacking 15/1 -> Mux/131
  Byte Unpacking 15/2 -> Mux/132
  Byte Unpacking 15/3 -> Mux/133
  Byte Unpacking 15/4 -> Mux/134
  Byte Unpacking 14/1 -> Mux/135
  Byte Unpacking 14/2 -> Mux/136
  Byte Unpacking 14/3 -> Mux/137
  Byte Unpacking 14/4 -> Mux/138
  Character C for check Sum3/1 -> Mux/139
  End of message 'L'3/1 -> Mux/140
  Constant34/1 -> Mux/141
  Constant35/1 -> Mux/142
  Constant31/1 -> Mux/143
  Constant3_2/1 -> Mux/144
  Embedded MATLAB Function2/1(hours) -> Mux/145
  Embedded MATLAB Function2/2(min) -> Mux/146
  Embedded MATLAB Function2/3(sec) -> Mux/147
  Embedded MATLAB Function2/4(date) -> Mux/148
  Embedded MATLAB Function2/5(month) -> Mux/149
  In1/1 -> Mux/154
  In2/1 -> Mux/155
  End of message 'L'4/1 -> Mux/153
  Character C for check Sum4/1 -> Mux/152
  Embedded MATLAB Function2/6(year) -> Byte Unpacking 16/1
  Byte Unpacking 16/1 -> Mux/150
  Byte Unpacking 16/2 -> Mux/151
  Data Type Conversion27/1 -> Byte Unpacking 1/1
  Data Type Conversion28/1 -> Byte Unpacking 2/1
  Data Type Conversion29/1 -> Byte Unpacking 5/1
  Data Type Conversion30/1 -> Byte Unpacking 3/1, Byte Unpacking 7/1, Byte Unpacking 12/1, Embedded MATLAB Function2/1(s)
  (m) to (cm)/1 -> Data Type Conversion27/1
  (m) to (cm)1/1 -> Data Type Conversion28/1
  (m) to (cm)2/1 -> Data Type Conversion29/1
  Vel_z/1 -> Data Type Conversion33/1
  Data Type Conversion33/1 -> Byte Unpacking 8/1
  Vel_y/1 -> Data Type Conversion32/1
  Data Type Conversion32/1 -> Byte Unpacking 6/1
  Vel_x/1 -> Data Type Conversion31/1
  Data Type Conversion31/1 -> Byte Unpacking 4/1
  Latitude/1 -> Data Type Conversion34/1
  Data Type Conversion34/1 -> Byte Unpacking 13/1
  Altitude/1 -> Data Type Conversion36/1
  Data Type Conversion36/1 -> Byte Unpacking 14/1
  "Longilitude "/1 -> Data Type Conversion35/1
  Data Type Conversion35/1 -> Byte Unpacking 15/1
  Mux/1 -> GPS/1

== system adcs_v15_integral_29april17/External Torques/Aerodynamic Torque ==
  v_Si : Inport
  x : Inport  Port=2
  Demux : Demux  Outputs=2
  aero torque : MATLAB Function  TreatAsAtomicUnit=on
  v_I to v_B : MATLAB Function  TreatAsAtomicUnit=on
  u_aero : Outport
  wires:
  v_I to v_B/1(v_B) -> aero torque/2(v_B)
  v_Si/1 -> Demux/1
  Demux/2 -> v_I to v_B/1(v_I)
  x/1 -> v_I to v_B/2(x)
  aero torque/1(u_aero) -> u_aero/1

== system adcs_v15_integral_29april17/External Torques/Subsystem ==
  v_Sun_b : Inport
  light : Inport  Port=2
  Solar_drag : MATLAB Function  TreatAsAtomicUnit=on
  Vector from CoM to CoP_in Body frame (yet to be finalized)2 : Constant  Value=v_COM_to_COP_b  VectorParams1D=off
  _ : aerolibutil/3x3 Cross Product
  u_Solar : Outport
  wires:
  _/1 -> u_Solar/1
  v_Sun_b/1 -> Solar_drag/1(v_Sun_b)
  light/1 -> Solar_drag/2(light)
  Solar_drag/1(solar_drag) -> _/2
  Vector from CoM to CoP_in Body frame (yet to be finalized)2/1 -> _/1

== system adcs_v15_integral_29april17/Sensors1/Magnetometer simple ==
  v_B_b : Inport
  Constant : Constant  Value=s_x_MAGMETER_BIAS
  Gaussian Noise Generator : commnoisgen2/Gaussian Noise Generator  m=0  d=s_x_MAGMETER  s=41  Ts=s_SIM_STEP_SIZE  frameBased=off  sampPerFrame=1  orient=off  outDataType=double
  Sum1 : Sum  Inputs=+++
  v_B_b(m) : Outport
  wires:
  Constant/1 -> Sum1/3
  Sum1/1 -> v_B_b(m)/1
  Gaussian Noise Generator/1 -> Sum1/1
  v_B_b/1 -> Sum1/2

== system adcs_v15_integral_29april17/Sensors1/Sun Sensors ==
  v_Sun_b : Inport
  Light : Inport  Port=2
  Embedded MATLAB Function : MATLAB Function  TreatAsAtomicUnit=on
  S1 : Subsystem
  S2 : Subsystem
  S3 : Subsystem
  S4 : Subsystem
  S5 : Subsystem
  S6 : Subsystem
  m_SUN : Outport
  wires:
  Embedded MATLAB Function/1(m_SUN) -> m_SUN/1
  v_Sun_b/1 -> S6/2(v_Sunb), S5/2(v_Sunb), S4/2(v_Sunb), S3/2(v_Sunb), S2/2(v_Sunb), S1/2(v_Sunb)
  S1/1(v_S) -> Embedded MATLAB Function/1(v_S1)
  S1/2(s_S) -> Embedded MATLAB Function/2(s_S1)
  S2/1(v_S) -> Embedded MATLAB Function/3(v_S2)
  S2/2(s_S) -> Embedded MATLAB Function/4(s_S2)
  S3/1(v_S) -> Embedded MATLAB Function/5(v_S3)
  S3/2(s_S) -> Embedded MATLAB Function/6(s_S3)
  S4/1(v_S) -> Embedded MATLAB Function/7(v_S4)
  S4/2(s_S) -> Embedded MATLAB Function/8(s_S4)
  S5/1(v_S) -> Embedded MATLAB Function/9(v_S5)
  S5/2(s_S) -> Embedded MATLAB Function/10(s_S5)
  S6/1(v_S) -> Embedded MATLAB Function/11(v_S6)
  S6/2(s_S) -> Embedded MATLAB Function/12(s_S6)
  Light/1 -> S1/1(light), S2/1(light), S3/1(light), S4/1(light), S5/1(light), S6/1(light)

== system adcs_v15_integral_29april17/Sensors2/Magnetometer simple ==
  v_B_b : Inport
  Constant : Constant  Value=s_x_MAGMETER_BIAS
  Gaussian Noise Generator : commnoisgen2/Gaussian Noise Generator  m=0  d=s_x_MAGMETER  s=41  Ts=s_SIM_STEP_SIZE  frameBased=off  sampPerFrame=1  orient=off  outDataType=double
  Sum1 : Sum  Inputs=+++
  v_B_b(m) : Outport
  wires:
  Constant/1 -> Sum1/3
  Sum1/1 -> v_B_b(m)/1
  Gaussian Noise Generator/1 -> Sum1/1
  v_B_b/1 -> Sum1/2

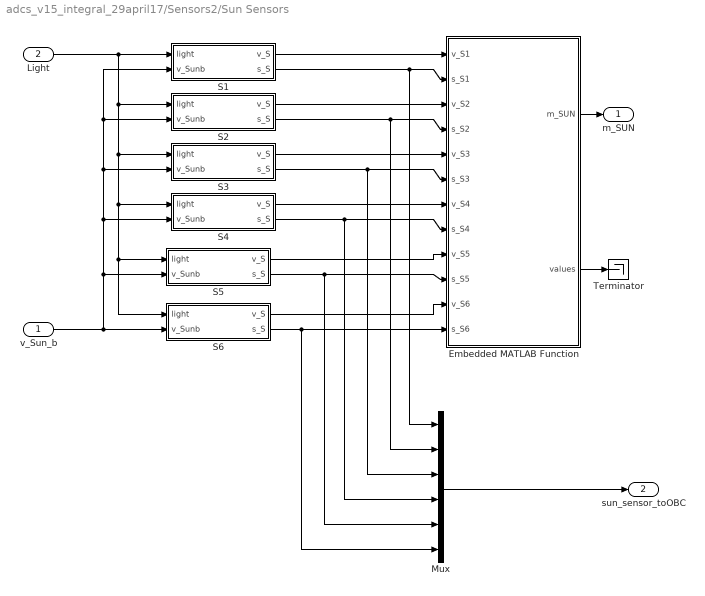
== system adcs_v15_integral_29april17/Sensors2/Sun Sensors ==
  v_Sun_b : Inport
  Light : Inport  Port=2
  Embedded MATLAB Function : MATLAB Function  TreatAsAtomicUnit=on
  Mux : Mux  Inputs=6
  S1 : Subsystem
  S2 : Subsystem
  S3 : Subsystem
  S4 : Subsystem
  S5 : Subsystem
  S6 : Subsystem
  Terminator : Terminator
  m_SUN : Outport
  sun_sensor_toOBC : Outport  Port=2
  wires:
  Embedded MATLAB Function/1(m_SUN) -> m_SUN/1
  v_Sun_b/1 -> S6/2(v_Sunb), S5/2(v_Sunb), S4/2(v_Sunb), S3/2(v_Sunb), S2/2(v_Sunb), S1/2(v_Sunb)
  S1/1(v_S) -> Embedded MATLAB Function/1(v_S1)
  S1/2(s_S) -> Mux/1, Embedded MATLAB Function/2(s_S1)
  S2/1(v_S) -> Embedded MATLAB Function/3(v_S2)
  S2/2(s_S) -> Mux/2, Embedded MATLAB Function/4(s_S2)
  S3/1(v_S) -> Embedded MATLAB Function/5(v_S3)
  S3/2(s_S) -> Mux/3, Embedded MATLAB Function/6(s_S3)
  S4/1(v_S) -> Embedded MATLAB Function/7(v_S4)
  S4/2(s_S) -> Mux/4, Embedded MATLAB Function/8(s_S4)
  S5/1(v_S) -> Embedded MATLAB Function/9(v_S5)
  S5/2(s_S) -> Mux/5, Embedded MATLAB Function/10(s_S5)
  S6/1(v_S) -> Embedded MATLAB Function/11(v_S6)
  S6/2(s_S) -> Mux/6, Embedded MATLAB Function/12(s_S6)
  Light/1 -> S1/1(light), S2/1(light), S3/1(light), S4/1(light), S5/1(light), S6/1(light)
  Mux/1 -> sun_sensor_toOBC/1
  Embedded MATLAB Function/2(values) -> Terminator/1

== system adcs_v15_integral_29april17/q -> w/Subsystem6 ==
  light : Inport
  (1-L) + L/z : MATLAB Function  TreatAsAtomicUnit=on
  Integer Delay : Delay  DelayLength=300  InputProcessing=Inherited
  Scope : Scope
  Scope1 : Scope
  Scope2 : Scope
  w-ctrl : Outport
  wires:
  (1-L) + L/z/1(y) -> Scope/1, w-ctrl/1
  light/1 -> (1-L) + L/z/1(a), Integer Delay/1, Scope2/1
  Integer Delay/1 -> Scope1/1, (1-L) + L/z/2(b)

== system adcs_v15_integral_29april17/Convert SGP to GPS/GPS/HDOP ==
  Data Type Conversion : DataTypeConversion  OutDataTypeStr=uint8
  Uniform Random Number : UniformRandomNumber  Minimum=0  Maximum=256  SampleTime=0.1
  Out1 : Outport
  wires:
  Uniform Random Number/1 -> Data Type Conversion/1
  Data Type Conversion/1 -> Out1/1

== system adcs_v15_integral_29april17/Convert SGP to GPS/GPS/HDOP1 ==
  Data Type Conversion : DataTypeConversion  OutDataTypeStr=uint8
  Uniform Random Number : UniformRandomNumber  Minimum=0  Maximum=256  SampleTime=0.1
  Out1 : Outport
  wires:
  Uniform Random Number/1 -> Data Type Conversion/1
  Data Type Conversion/1 -> Out1/1

== system adcs_v15_integral_29april17/Convert SGP to GPS/GPS/random uint1 ==
  Data Type Conversion : DataTypeConversion  OutDataTypeStr=uint8
  Uniform Random Number : UniformRandomNumber  Minimum=0  Maximum=256  SampleTime=0.1
  Out1 : Outport
  wires:
  Uniform Random Number/1 -> Data Type Conversion/1
  Data Type Conversion/1 -> Out1/1

== system adcs_v15_integral_29april17/Convert SGP to GPS/GPS/random uint2 ==
  Data Type Conversion : DataTypeConversion  OutDataTypeStr=uint8
  Uniform Random Number : UniformRandomNumber  Minimum=0  Maximum=256  SampleTime=0.1
  Out1 : Outport
  wires:
  Uniform Random Number/1 -> Data Type Conversion/1
  Data Type Conversion/1 -> Out1/1

== system adcs_v15_integral_29april17/Convert SGP to GPS/GPS/random uint3 ==
  Data Type Conversion : DataTypeConversion  OutDataTypeStr=uint8
  Uniform Random Number : UniformRandomNumber  Minimum=0  Maximum=256  SampleTime=0.1
  Out1 : Outport
  wires:
  Uniform Random Number/1 -> Data Type Conversion/1
  Data Type Conversion/1 -> Out1/1

== system adcs_v15_integral_29april17/Convert SGP to GPS/GPS/random uint4 ==
  Data Type Conversion : DataTypeConversion  OutDataTypeStr=uint8
  Uniform Random Number : UniformRandomNumber  Minimum=0  Maximum=256  SampleTime=0.1
  Out1 : Outport
  wires:
  Uniform Random Number/1 -> Data Type Conversion/1
  Data Type Conversion/1 -> Out1/1

== system adcs_v15_integral_29april17/Convert SGP to GPS/GPS/random uint5 ==
  Data Type Conversion : DataTypeConversion  OutDataTypeStr=uint8
  Uniform Random Number : UniformRandomNumber  Minimum=0  Maximum=256  SampleTime=0.1
  Out1 : Outport
  wires:
  Uniform Random Number/1 -> Data Type Conversion/1
  Data Type Conversion/1 -> Out1/1

== system adcs_v15_integral_29april17/Convert SGP to GPS/GPS/random uint6 ==
  Data Type Conversion : DataTypeConversion  OutDataTypeStr=uint8
  Uniform Random Number : UniformRandomNumber  Minimum=0  Maximum=256  SampleTime=0.1
  Out1 : Outport
  wires:
  Uniform Random Number/1 -> Data Type Conversion/1
  Data Type Conversion/1 -> Out1/1

== system adcs_v15_integral_29april17/Convert SGP to GPS/GPS/random uint7 ==
  Data Type Conversion : DataTypeConversion  OutDataTypeStr=uint8
  Uniform Random Number : UniformRandomNumber  Minimum=0  Maximum=256  SampleTime=0.1
  Out1 : Outport
  wires:
  Uniform Random Number/1 -> Data Type Conversion/1
  Data Type Conversion/1 -> Out1/1

== system adcs_v15_integral_29april17/Convert SGP to GPS/GPS/random uint8 ==
  Data Type Conversion : DataTypeConversion  OutDataTypeStr=uint8
  Uniform Random Number : UniformRandomNumber  Minimum=0  Maximum=256  SampleTime=0.1
  Out1 : Outport
  wires:
  Uniform Random Number/1 -> Data Type Conversion/1
  Data Type Conversion/1 -> Out1/1

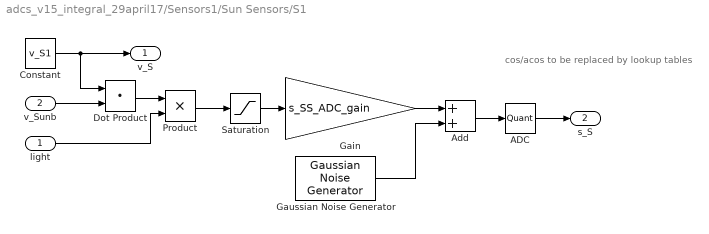
== system adcs_v15_integral_29april17/Sensors1/Sun Sensors/S1 ==
  note: cos/acos to be replaced by lookup tables
  light : Inport
  v_Sunb : Inport  Port=2
  ADC : Quantizer  QuantizationInterval=1/s_SS_ADC_res
  Add : Sum
  Constant : Constant  Value=v_S1
  Dot Product : DotProduct  InputSameDT=on  OutDataTypeStr=Inherit: Inherit via internal rule
  Gain : Gain  Gain=s_SS_ADC_gain
  Gaussian Noise Generator : commnoisgen2/Gaussian Noise Generator  m=0  d=s_x_SUNSENSOR  s=41  Ts=s_SIM_STEP_SIZE  frameBased=off  sampPerFrame=1  orient=off  outDataType=double
  Product : Product  RndMeth=Zero
  Saturation : Saturate  UpperLimit=inf  LowerLimit=0
  v_S : Outport
  s_S : Outport  Port=2
  wires:
  light/1 -> Product/2
  Product/1 -> Saturation/1
  Dot Product/1 -> Product/1
  v_Sunb/1 -> Dot Product/2
  Saturation/1 -> Gain/1
  Constant/1 -> v_S/1, Dot Product/1
  Gaussian Noise Generator/1 -> Add/2
  Gain/1 -> Add/1
  Add/1 -> ADC/1
  ADC/1 -> s_S/1

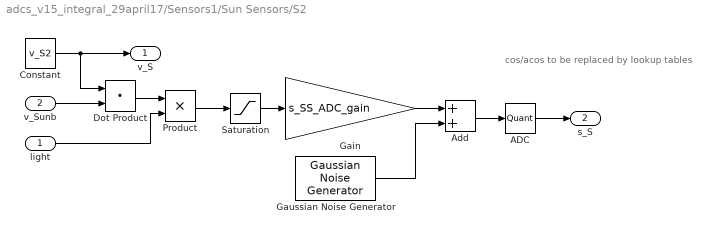
== system adcs_v15_integral_29april17/Sensors1/Sun Sensors/S2 ==
  note: cos/acos to be replaced by lookup tables
  light : Inport
  v_Sunb : Inport  Port=2
  ADC : Quantizer  QuantizationInterval=1/s_SS_ADC_res
  Add : Sum
  Constant : Constant  Value=v_S2
  Dot Product : DotProduct  InputSameDT=on  OutDataTypeStr=Inherit: Inherit via internal rule
  Gain : Gain  Gain=s_SS_ADC_gain
  Gaussian Noise Generator : commnoisgen2/Gaussian Noise Generator  m=0  d=s_x_SUNSENSOR  s=41  Ts=s_SIM_STEP_SIZE  frameBased=off  sampPerFrame=1  orient=off  outDataType=double
  Product : Product  RndMeth=Zero
  Saturation : Saturate  UpperLimit=inf  LowerLimit=0
  v_S : Outport
  s_S : Outport  Port=2
  wires:
  ADC/1 -> s_S/1
  Add/1 -> ADC/1
  Gain/1 -> Add/1
  Gaussian Noise Generator/1 -> Add/2
  Constant/1 -> Dot Product/1, v_S/1
  Saturation/1 -> Gain/1
  v_Sunb/1 -> Dot Product/2
  Dot Product/1 -> Product/1
  Product/1 -> Saturation/1
  light/1 -> Product/2

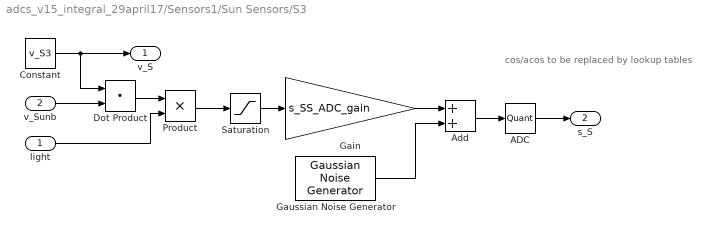
== system adcs_v15_integral_29april17/Sensors1/Sun Sensors/S3 ==
  note: cos/acos to be replaced by lookup tables
  light : Inport
  v_Sunb : Inport  Port=2
  ADC : Quantizer  QuantizationInterval=1/s_SS_ADC_res
  Add : Sum
  Constant : Constant  Value=v_S3
  Dot Product : DotProduct  InputSameDT=on  OutDataTypeStr=Inherit: Inherit via internal rule
  Gain : Gain  Gain=s_SS_ADC_gain
  Gaussian Noise Generator : commnoisgen2/Gaussian Noise Generator  m=0  d=s_x_SUNSENSOR  s=41  Ts=s_SIM_STEP_SIZE  frameBased=off  sampPerFrame=1  orient=off  outDataType=double
  Product : Product  RndMeth=Zero
  Saturation : Saturate  UpperLimit=inf  LowerLimit=0
  v_S : Outport
  s_S : Outport  Port=2
  wires:
  light/1 -> Product/2
  Product/1 -> Saturation/1
  Dot Product/1 -> Product/1
  v_Sunb/1 -> Dot Product/2
  Saturation/1 -> Gain/1
  Constant/1 -> v_S/1, Dot Product/1
  Gaussian Noise Generator/1 -> Add/2
  Gain/1 -> Add/1
  Add/1 -> ADC/1
  ADC/1 -> s_S/1

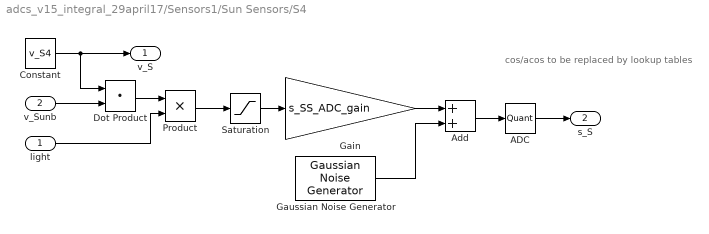
== system adcs_v15_integral_29april17/Sensors1/Sun Sensors/S4 ==
  note: cos/acos to be replaced by lookup tables
  light : Inport
  v_Sunb : Inport  Port=2
  ADC : Quantizer  QuantizationInterval=1/s_SS_ADC_res
  Add : Sum
  Constant : Constant  Value=v_S4
  Dot Product : DotProduct  InputSameDT=on  OutDataTypeStr=Inherit: Inherit via internal rule
  Gain : Gain  Gain=s_SS_ADC_gain
  Gaussian Noise Generator : commnoisgen2/Gaussian Noise Generator  m=0  d=s_x_SUNSENSOR  s=41  Ts=s_SIM_STEP_SIZE  frameBased=off  sampPerFrame=1  orient=off  outDataType=double
  Product : Product  RndMeth=Zero
  Saturation : Saturate  UpperLimit=inf  LowerLimit=0
  v_S : Outport
  s_S : Outport  Port=2
  wires:
  ADC/1 -> s_S/1
  Add/1 -> ADC/1
  Gain/1 -> Add/1
  Gaussian Noise Generator/1 -> Add/2
  Constant/1 -> Dot Product/1, v_S/1
  Saturation/1 -> Gain/1
  v_Sunb/1 -> Dot Product/2
  Dot Product/1 -> Product/1
  Product/1 -> Saturation/1
  light/1 -> Product/2

== system adcs_v15_integral_29april17/Sensors1/Sun Sensors/S5 ==
  note: cos/acos to be replaced by lookup tables
  light : Inport
  v_Sunb : Inport  Port=2
  ADC : Quantizer  QuantizationInterval=1/s_SS_ADC_res
  Add : Sum
  Constant : Constant  Value=v_S5
  Dot Product : DotProduct  InputSameDT=on  OutDataTypeStr=Inherit: Inherit via internal rule
  Gain : Gain  Gain=s_SS_ADC_gain
  Gaussian Noise Generator : commnoisgen2/Gaussian Noise Generator  m=0  d=s_x_SUNSENSOR  s=41  Ts=s_SIM_STEP_SIZE  frameBased=off  sampPerFrame=1  orient=off  outDataType=double
  Product : Product  RndMeth=Zero
  Saturation : Saturate  UpperLimit=inf  LowerLimit=0
  v_S : Outport
  s_S : Outport  Port=2
  wires:
  light/1 -> Product/2
  Product/1 -> Saturation/1
  Dot Product/1 -> Product/1
  v_Sunb/1 -> Dot Product/2
  Saturation/1 -> Gain/1
  Constant/1 -> v_S/1, Dot Product/1
  Gaussian Noise Generator/1 -> Add/2
  Gain/1 -> Add/1
  Add/1 -> ADC/1
  ADC/1 -> s_S/1

== system adcs_v15_integral_29april17/Sensors1/Sun Sensors/S6 ==
  note: cos/acos to be replaced by lookup tables
  light : Inport
  v_Sunb : Inport  Port=2
  ADC : Quantizer  QuantizationInterval=1/s_SS_ADC_res
  Add : Sum
  Constant : Constant  Value=v_S6
  Dot Product : DotProduct  InputSameDT=on  OutDataTypeStr=Inherit: Inherit via internal rule
  Gain : Gain  Gain=s_SS_ADC_gain
  Gaussian Noise Generator : commnoisgen2/Gaussian Noise Generator  m=0  d=s_x_SUNSENSOR  s=41  Ts=s_SIM_STEP_SIZE  frameBased=off  sampPerFrame=1  orient=off  outDataType=double
  Product : Product  RndMeth=Zero
  Saturation : Saturate  UpperLimit=inf  LowerLimit=0
  v_S : Outport
  s_S : Outport  Port=2
  wires:
  ADC/1 -> s_S/1
  Add/1 -> ADC/1
  Gain/1 -> Add/1
  Gaussian Noise Generator/1 -> Add/2
  Constant/1 -> Dot Product/1, v_S/1
  Saturation/1 -> Gain/1
  v_Sunb/1 -> Dot Product/2
  Dot Product/1 -> Product/1
  Product/1 -> Saturation/1
  light/1 -> Product/2
